simulink model "ML3phase"  (R2021a)
settings: Solver=VariableStepAuto  StartTime=0.0  StopTime=0.4  RelTol=1e-3
InitFcn:
  | alp1=30;
  | alp2=60;
values from neighbouring files (symbols this model uses):
  Alpha1 = z(1)    [ML3ph.m]
  Alpha2 = z(2)    [ML3ph.m]
  Alpha3 = z(3)    [ML3ph.m]
libraries: spsMosfetLib x36, spsCurrentMeasurementLib x10, spsDCVoltageSourceLib x9, spspowerguiLib x4, spsVoltageMeasurementLib x3, spsSeriesRLCBranchLib x3, spsGroundLib x1, spsRMSLib x1, spsThreePhaseVIMeasurementLib x1
settings Model: Creator=oem  LastModifiedBy=Islam
settings SolverCC: AlgebraicLoopSolver=TrustRegion
settings DataIOCC: SignalLogging=off  DSMLogging=off  ReturnWorkspaceOutputs=off
settings OptimizationCC: LifeSpan=inf
settings DebuggingCC: UnconnectedInputMsg=none  UnconnectedOutputMsg=none  UnconnectedLineMsg=none  SFMachineParentedDataDiag=warning  ArithmeticOperatorsInVariantConditions=warning
settings ModelReferenceCC: EnableRefExpFcnMdlSchedulingChecks=off
settings SFSimCC: CustomCodeUndefinedFunction=UseInterfaceOnly
settings RTWCC: Description=Generic Real-Time Target
settings CodeAppCC: StateflowObjectComments=on

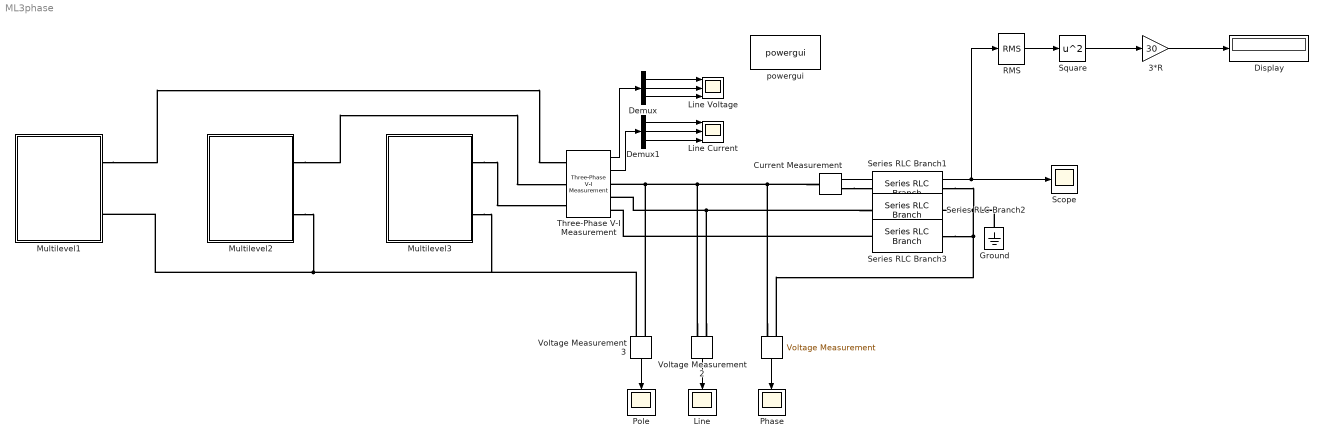
== system ML3phase ==
  " " : spsVoltageMeasurementLib/Voltage Measurement  PhasorSimulation=off  OutputType=Complex  PSBequivalent=0
  3*R : Gain  Gain=30
  Current Measurement : spsCurrentMeasurementLib/Current Measurement  PhasorSimulation=off  OutputType=Complex  PSBequivalent=0
  Demux : Demux  Outputs=3
  Demux1 : Demux  Outputs=3
  Display : Display
  Ground : spsGroundLib/Ground  LConnTagsString=a
  Line : Scope
  Line Current : Scope  NumInputPorts=3
  Line Voltage : Scope  NumInputPorts=3
  Multilevel1 : Subsystem
  Multilevel2 : Subsystem
  Multilevel3 : Subsystem
  Phase : Scope
  Pole : Scope
  RMS : spsRMSLib/RMS  TrueRMS=on  Freq=50  RMSInit=0  Ts=0
  Scope : Scope
  Series RLC Branch1 : spsSeriesRLCBranchLib/Series RLC Branch  LConnTagsString=__new0  RConnTagsString=__new0  BranchType=RL  Resistance=10  Inductance=1e-3  SetiL0=off  InitialCurrent=0  Capacitance=1e-6  Setx0=off  InitialVoltage=0  Measurements=None
  Series RLC Branch2 : spsSeriesRLCBranchLib/Series RLC Branch  LConnTagsString=__new0  RConnTagsString=__new0  BranchType=RL  Resistance=10  Inductance=1e-3  SetiL0=off  InitialCurrent=0  Capacitance=1e-6  Setx0=off  InitialVoltage=0  Measurements=None
  Series RLC Branch3 : spsSeriesRLCBranchLib/Series RLC Branch  LConnTagsString=__new0  RConnTagsString=__new0  BranchType=RL  Resistance=10  Inductance=1e-3  SetiL0=off  InitialCurrent=0  Capacitance=1e-6  Setx0=off  InitialVoltage=0  Measurements=None
  Square : Math  Operator=square  SaturateOnIntegerOverflow=on
  Three-Phase V-I Measurement : spsThreePhaseVIMeasurementLib/Three-Phase V-I Measurement  VoltageMeasurement=phase-to-phase  SetLabelV=off  LabelV=Vabc  Vpu=off  VpuLL=off  CurrentMeasurement=yes  SetLabelI=off  LabelI=Iabc  Ipu=off  Pbase=100e6  Vbase=500e3  OutputType=Complex  PhasorSimulation=off  PSBequivalent=0
  Voltage Measurement2 : spsVoltageMeasurementLib/Voltage Measurement  PhasorSimulation=off  OutputType=Complex  PSBequivalent=0
  Voltage Measurement3 : spsVoltageMeasurementLib/Voltage Measurement  PhasorSimulation=off  OutputType=Complex  PSBequivalent=0
  powergui : spspowerguiLib/powergui  Priority=1  SimulationMode=Continuous  SampleTime=50e-6  frequency=60  Iterations=50  frequencyindice=0  Pbase=100e6  ErrMax=1e-4  UnitsV=kV  UnitsW=MW  buscounter=0  FunctionMessages=off  echomessages=off  EnableUseOfTLC=off  CurrentSourceSwitches=off  DisableSnubberDevices=off  DisableRonSwitches=off  DisableVfSwitches=off  DisplayEquations=off  AutomaticDiscreteSolvers=off  SolverType=Tustin/Backward Euler (TBE)  Interpol=off  ExternalGateDelay=off  methode=off  Ts=100  x0status=blocks  SPID=on  SwTol=0  HookPort=off  NonlinearTolerance=1e-4  nMaxIteration=100  ContinueOnMaxIteration=off  RestoreLinks=warning  ResistiveCurrentMeasurement=off  Frange=[0:2:500]  Ylog=off  Xlog=on  ShowGrid=off  save=off  variable=ZData  structure=0  ZoomFFT=off  StartTime=0.0  cycles=1  DisplayStyle=1  fundamental=60  FreqAxis=off  MaxFrequency=1000  frequencyindicesteady=1  RmsSteady=1  display=off
  wires:
  Demux/3 -> Line Voltage/3
  Demux/1 -> Line Voltage/1
  Three-Phase V-I Measurement/1 -> Demux/1
  Demux/2 -> Line Voltage/2
  Demux1/1 -> Line Current/1
  Demux1/3 -> Line Current/3
  Three-Phase V-I Measurement/2 -> Demux1/1
  Demux1/2 -> Line Current/2
  " "/1 -> Phase/1
  Voltage Measurement2/1 -> Line/1
  Voltage Measurement3/1 -> Pole/1
  Current Measurement/1 -> RMS/1, Scope/1
  RMS/1 -> Square/1
  Square/1 -> 3*R/1
  3*R/1 -> Display/1
  connections:
  Multilevel2/RConn2 -- Voltage Measurement3/LConn2 -- Multilevel3/RConn2 -- Multilevel1/RConn2
  Multilevel3/RConn1 -- Three-Phase V-I Measurement/LConn3
  Multilevel2/RConn1 -- Three-Phase V-I Measurement/LConn2
  Multilevel1/RConn1 -- Three-Phase V-I Measurement/LConn1
  Series RLC Branch3/RConn1 -- Series RLC Branch2/RConn1 -- Series RLC Branch1/RConn1 -- Ground/LConn1 -- " "/LConn2
  " "/LConn1 -- Voltage Measurement2/LConn1 -- Voltage Measurement3/LConn1 -- Three-Phase V-I Measurement/RConn1 -- Current Measurement/LConn1
  Series RLC Branch2/LConn1 -- Voltage Measurement2/LConn2 -- Three-Phase V-I Measurement/RConn2
  Series RLC Branch3/LConn1 -- Three-Phase V-I Measurement/RConn3
  Current Measurement/RConn1 -- Series RLC Branch1/LConn1

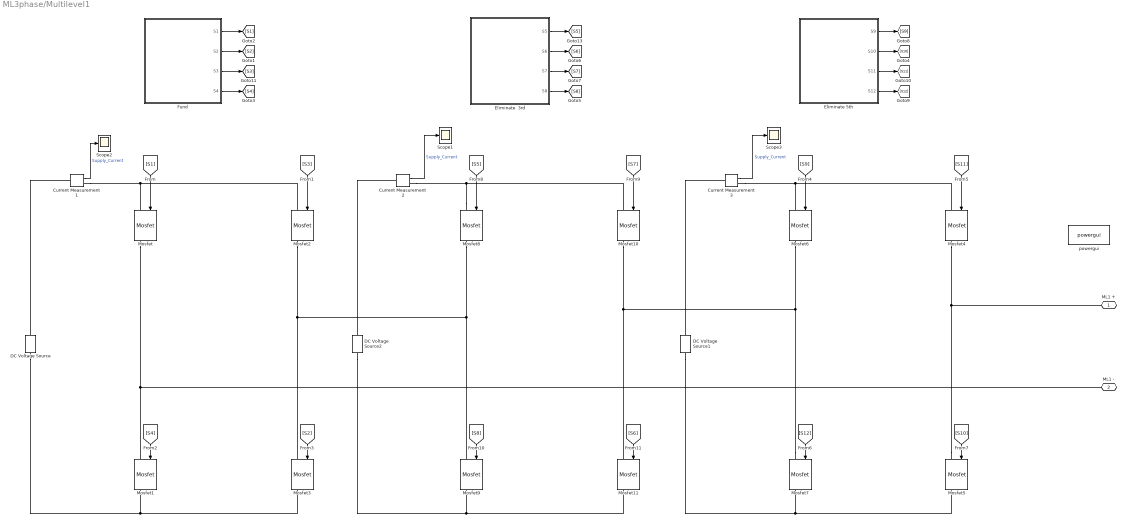
== system ML3phase/Multilevel1 ==
  Current Measurement1 : spsCurrentMeasurementLib/Current Measurement  PhasorSimulation=off  OutputType=Complex  PSBequivalent=0
  Current Measurement2 : spsCurrentMeasurementLib/Current Measurement  PhasorSimulation=off  OutputType=Complex  PSBequivalent=0
  Current Measurement3 : spsCurrentMeasurementLib/Current Measurement  PhasorSimulation=off  OutputType=Complex  PSBequivalent=0
  DC Voltage Source : spsDCVoltageSourceLib/DC Voltage Source  Amplitude=200/3  Measurements=Voltage
  DC Voltage Source1 : spsDCVoltageSourceLib/DC Voltage Source  Amplitude=200/3  Measurements=Voltage
  DC Voltage Source2 : spsDCVoltageSourceLib/DC Voltage Source  Amplitude=200/3  Measurements=Voltage
  Eliminate  3rd : Subsystem
  Eliminate 5th : Subsystem
  Fund : Subsystem
  Mosfet{,1..11} (12 alike) : spsMosfetLib/Mosfet  Ron=0.1  Lon=0  Rd=0.01  Vfd=0  IC=0  Rs=1e5  Cs=inf  Measurements=on
  Scope1 : Scope
  Scope2 : Scope
  Scope3 : Scope
  powergui : spspowerguiLib/powergui  Priority=1  SimulationMode=Continuous  SampleTime=1e-6  frequency=60  Iterations=50  frequencyindice=0  Pbase=100e6  ErrMax=1e-4  UnitsV=kV  UnitsW=MW  buscounter=0  FunctionMessages=off  echomessages=off  EnableUseOfTLC=off  CurrentSourceSwitches=off  DisableSnubberDevices=off  DisableRonSwitches=off  DisableVfSwitches=off  DisplayEquations=off  AutomaticDiscreteSolvers=off  SolverType=Tustin/Backward Euler (TBE)  Interpol=off  ExternalGateDelay=off  methode=off  Ts=100  x0status=blocks  SPID=on  SwTol=0  HookPort=off  NonlinearTolerance=1e-4  nMaxIteration=100  ContinueOnMaxIteration=off  RestoreLinks=warning  ResistiveCurrentMeasurement=off  Frange=[0:2:500]  Ylog=off  Xlog=on  ShowGrid=off  save=off  variable=ZData  structure=0  ZoomFFT=off  StartTime=0.0  cycles=1  DisplayStyle=1  fundamental=60  FreqAxis=off  MaxFrequency=1000  frequencyindicesteady=1  RmsSteady=1  display=off
  "ML1 + " : PMIOPort  Side=Right
  ML1 - : PMIOPort  Port=2  Side=Right
  wires:
  Eliminate 5th/1(S9) -> [S9]
  Fund/1(S1) -> [S1]
  [S8] -> Mosfet9/1
  [S1] -> Mosfet/1
  Eliminate  3rd/2(S6) -> [S6]
  [S12] -> Mosfet7/1
  [S11] -> Mosfet4/1
  Current Measurement3/1 -> Scope3/1  "Supply_Current"
  Eliminate 5th/2(S10) -> [S10]
  Fund/3(S3) -> [S3]
  [S2] -> Mosfet3/1
  Eliminate  3rd/1(S5) -> [S5]
  [S3] -> Mosfet2/1
  Current Measurement2/1 -> Scope1/1  "Supply_Current"
  Fund/2(S2) -> [S2]
  Current Measurement1/1 -> Scope2/1  "Supply_Current"
  [S4] -> Mosfet1/1
  [S5] -> Mosfet8/1
  [S6] -> Mosfet11/1
  Eliminate 5th/3(S11) -> [S11]
  Fund/4(S4) -> [S4]
  [S10] -> Mosfet5/1
  [S7] -> Mosfet10/1
  [S9] -> Mosfet6/1
  Eliminate  3rd/4(S8) -> [S8]
  Eliminate  3rd/3(S7) -> [S7]
  Eliminate 5th/4(S12) -> [S12]
  connections:
  Mosfet11/RConn1 -- DC Voltage Source2/LConn1 -- Mosfet9/RConn1
  Mosfet1/RConn1 -- Mosfet3/RConn1 -- DC Voltage Source/LConn1
  Mosfet8/LConn1 -- Current Measurement2/RConn1 -- Mosfet10/LConn1
  Mosfet5/LConn1 -- "ML1 + "/RConn1 -- Mosfet4/RConn1
  Current Measurement1/RConn1 -- Mosfet/LConn1 -- Mosfet2/LConn1
  Mosfet7/LConn1 -- Mosfet6/RConn1 -- Mosfet11/LConn1 -- Mosfet10/RConn1
  DC Voltage Source1/LConn1 -- Mosfet5/RConn1 -- Mosfet7/RConn1
  Mosfet/RConn1 -- Mosfet1/LConn1 -- ML1 -/RConn1
  Mosfet8/RConn1 -- Mosfet9/LConn1 -- Mosfet2/RConn1 -- Mosfet3/LConn1
  Current Measurement3/RConn1 -- Mosfet6/LConn1 -- Mosfet4/LConn1
  Current Measurement2/LConn1 -- DC Voltage Source2/RConn1
  Current Measurement3/LConn1 -- DC Voltage Source1/RConn1
  Current Measurement1/LConn1 -- DC Voltage Source/RConn1

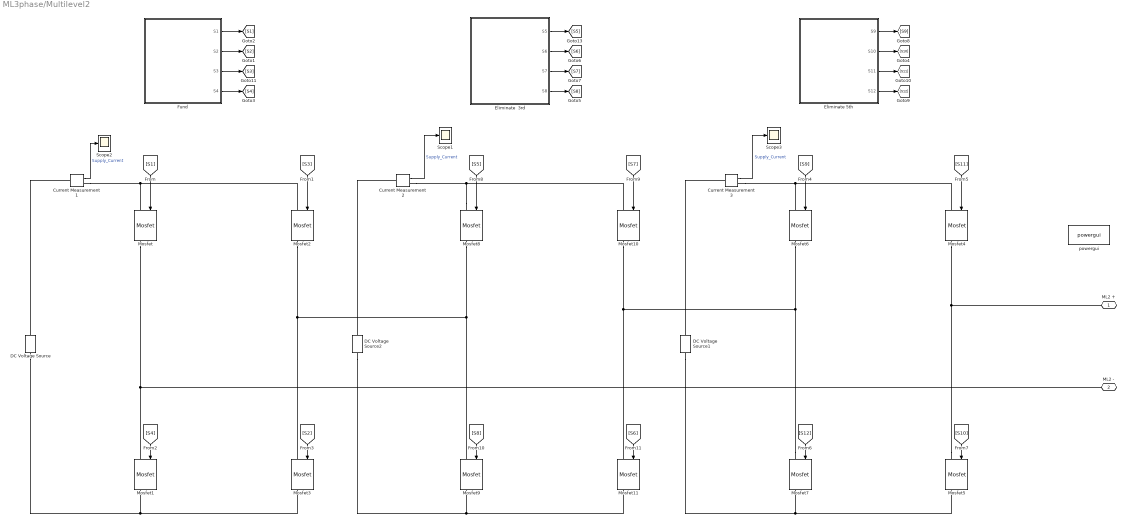
== system ML3phase/Multilevel2 ==
  Current Measurement1 : spsCurrentMeasurementLib/Current Measurement  PhasorSimulation=off  OutputType=Complex  PSBequivalent=0
  Current Measurement2 : spsCurrentMeasurementLib/Current Measurement  PhasorSimulation=off  OutputType=Complex  PSBequivalent=0
  Current Measurement3 : spsCurrentMeasurementLib/Current Measurement  PhasorSimulation=off  OutputType=Complex  PSBequivalent=0
  DC Voltage Source : spsDCVoltageSourceLib/DC Voltage Source  Amplitude=200/3  Measurements=Voltage
  DC Voltage Source1 : spsDCVoltageSourceLib/DC Voltage Source  Amplitude=200/3  Measurements=Voltage
  DC Voltage Source2 : spsDCVoltageSourceLib/DC Voltage Source  Amplitude=200/3  Measurements=Voltage
  Eliminate  3rd : Subsystem
  Eliminate 5th : Subsystem
  Fund : Subsystem
  Mosfet{,1..11} (12 alike) : spsMosfetLib/Mosfet  Ron=0.1  Lon=0  Rd=0.01  Vfd=0  IC=0  Rs=1e5  Cs=inf  Measurements=on
  Scope1 : Scope
  Scope2 : Scope
  Scope3 : Scope
  powergui : spspowerguiLib/powergui  Priority=1  SimulationMode=Continuous  SampleTime=1e-6  frequency=60  Iterations=50  frequencyindice=0  Pbase=100e6  ErrMax=1e-4  UnitsV=kV  UnitsW=MW  buscounter=0  FunctionMessages=off  echomessages=off  EnableUseOfTLC=off  CurrentSourceSwitches=off  DisableSnubberDevices=off  DisableRonSwitches=off  DisableVfSwitches=off  DisplayEquations=off  AutomaticDiscreteSolvers=off  SolverType=Tustin/Backward Euler (TBE)  Interpol=off  ExternalGateDelay=off  methode=off  Ts=100  x0status=blocks  SPID=on  SwTol=0  HookPort=off  NonlinearTolerance=1e-4  nMaxIteration=100  ContinueOnMaxIteration=off  RestoreLinks=warning  ResistiveCurrentMeasurement=off  Frange=[0:2:500]  Ylog=off  Xlog=on  ShowGrid=off  save=off  variable=ZData  structure=0  ZoomFFT=off  StartTime=0.0  cycles=1  DisplayStyle=1  fundamental=60  FreqAxis=off  MaxFrequency=1000  frequencyindicesteady=1  RmsSteady=1  display=off
  "ML2 + " : PMIOPort  Side=Right
  ML2 - : PMIOPort  Port=2  Side=Right
  wires:
  Eliminate 5th/1(S9) -> [S9]
  Fund/1(S1) -> [S1]
  [S8] -> Mosfet9/1
  [S1] -> Mosfet/1
  Eliminate  3rd/2(S6) -> [S6]
  [S12] -> Mosfet7/1
  [S11] -> Mosfet4/1
  Current Measurement3/1 -> Scope3/1  "Supply_Current"
  Eliminate 5th/2(S10) -> [S10]
  Fund/3(S3) -> [S3]
  [S2] -> Mosfet3/1
  Eliminate  3rd/1(S5) -> [S5]
  [S3] -> Mosfet2/1
  Current Measurement2/1 -> Scope1/1  "Supply_Current"
  Fund/2(S2) -> [S2]
  Current Measurement1/1 -> Scope2/1  "Supply_Current"
  [S4] -> Mosfet1/1
  [S5] -> Mosfet8/1
  [S6] -> Mosfet11/1
  Eliminate 5th/3(S11) -> [S11]
  Fund/4(S4) -> [S4]
  [S10] -> Mosfet5/1
  [S7] -> Mosfet10/1
  [S9] -> Mosfet6/1
  Eliminate  3rd/4(S8) -> [S8]
  Eliminate  3rd/3(S7) -> [S7]
  Eliminate 5th/4(S12) -> [S12]
  connections:
  Mosfet11/RConn1 -- DC Voltage Source2/LConn1 -- Mosfet9/RConn1
  Mosfet1/RConn1 -- Mosfet3/RConn1 -- DC Voltage Source/LConn1
  Mosfet8/LConn1 -- Current Measurement2/RConn1 -- Mosfet10/LConn1
  Mosfet5/LConn1 -- Mosfet4/RConn1 -- "ML2 + "/RConn1
  Current Measurement1/RConn1 -- Mosfet/LConn1 -- Mosfet2/LConn1
  Mosfet7/LConn1 -- Mosfet6/RConn1 -- Mosfet11/LConn1 -- Mosfet10/RConn1
  DC Voltage Source1/LConn1 -- Mosfet5/RConn1 -- Mosfet7/RConn1
  ML2 -/RConn1 -- Mosfet/RConn1 -- Mosfet1/LConn1
  Mosfet8/RConn1 -- Mosfet9/LConn1 -- Mosfet2/RConn1 -- Mosfet3/LConn1
  Current Measurement3/RConn1 -- Mosfet6/LConn1 -- Mosfet4/LConn1
  Current Measurement2/LConn1 -- DC Voltage Source2/RConn1
  Current Measurement3/LConn1 -- DC Voltage Source1/RConn1
  Current Measurement1/LConn1 -- DC Voltage Source/RConn1

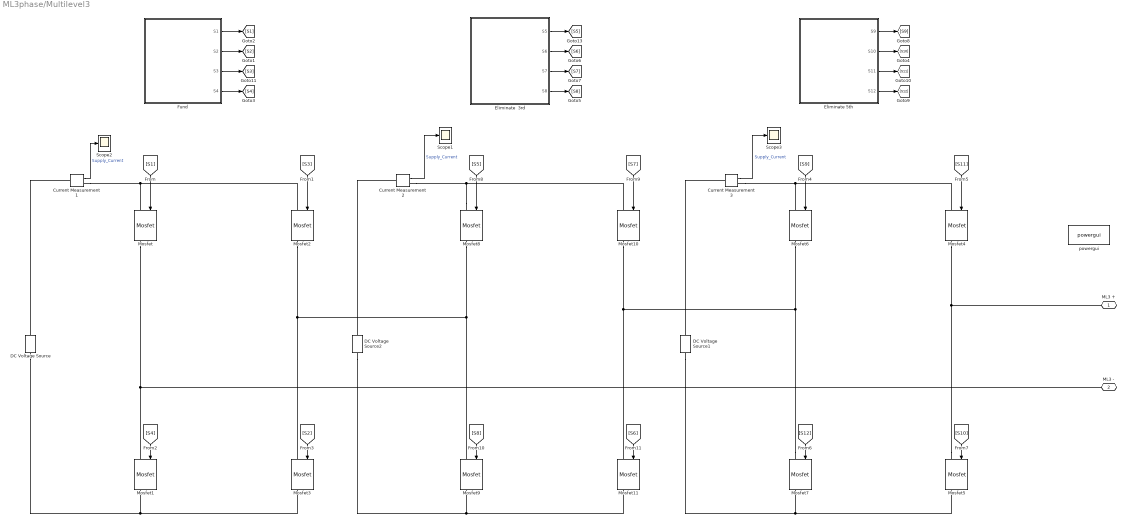
== system ML3phase/Multilevel3 ==
  Current Measurement1 : spsCurrentMeasurementLib/Current Measurement  PhasorSimulation=off  OutputType=Complex  PSBequivalent=0
  Current Measurement2 : spsCurrentMeasurementLib/Current Measurement  PhasorSimulation=off  OutputType=Complex  PSBequivalent=0
  Current Measurement3 : spsCurrentMeasurementLib/Current Measurement  PhasorSimulation=off  OutputType=Complex  PSBequivalent=0
  DC Voltage Source : spsDCVoltageSourceLib/DC Voltage Source  Amplitude=200/3  Measurements=Voltage
  DC Voltage Source1 : spsDCVoltageSourceLib/DC Voltage Source  Amplitude=200/3  Measurements=Voltage
  DC Voltage Source2 : spsDCVoltageSourceLib/DC Voltage Source  Amplitude=200/3  Measurements=Voltage
  Eliminate  3rd : Subsystem
  Eliminate 5th : Subsystem
  Fund : Subsystem
  Mosfet{,1..11} (12 alike) : spsMosfetLib/Mosfet  Ron=0.1  Lon=0  Rd=0.01  Vfd=0  IC=0  Rs=1e5  Cs=inf  Measurements=on
  Scope1 : Scope
  Scope2 : Scope
  Scope3 : Scope
  powergui : spspowerguiLib/powergui  Priority=1  SimulationMode=Continuous  SampleTime=1e-6  frequency=60  Iterations=50  frequencyindice=0  Pbase=100e6  ErrMax=1e-4  UnitsV=kV  UnitsW=MW  buscounter=0  FunctionMessages=off  echomessages=off  EnableUseOfTLC=off  CurrentSourceSwitches=off  DisableSnubberDevices=off  DisableRonSwitches=off  DisableVfSwitches=off  DisplayEquations=off  AutomaticDiscreteSolvers=off  SolverType=Tustin/Backward Euler (TBE)  Interpol=off  ExternalGateDelay=off  methode=off  Ts=100  x0status=blocks  SPID=on  SwTol=0  HookPort=off  NonlinearTolerance=1e-4  nMaxIteration=100  ContinueOnMaxIteration=off  RestoreLinks=warning  ResistiveCurrentMeasurement=off  Frange=[0:2:500]  Ylog=off  Xlog=on  ShowGrid=off  save=off  variable=ZData  structure=0  ZoomFFT=off  StartTime=0.0  cycles=1  DisplayStyle=1  fundamental=60  FreqAxis=off  MaxFrequency=1000  frequencyindicesteady=1  RmsSteady=1  display=off
  "ML3 + " : PMIOPort  Side=Right
  ML3 - : PMIOPort  Port=2  Side=Right
  wires:
  Eliminate 5th/1(S9) -> [S9]
  Fund/1(S1) -> [S1]
  [S8] -> Mosfet9/1
  [S1] -> Mosfet/1
  Eliminate  3rd/2(S6) -> [S6]
  [S12] -> Mosfet7/1
  [S11] -> Mosfet4/1
  Current Measurement3/1 -> Scope3/1  "Supply_Current"
  Eliminate 5th/2(S10) -> [S10]
  Fund/3(S3) -> [S3]
  [S2] -> Mosfet3/1
  Eliminate  3rd/1(S5) -> [S5]
  [S3] -> Mosfet2/1
  Current Measurement2/1 -> Scope1/1  "Supply_Current"
  Fund/2(S2) -> [S2]
  Current Measurement1/1 -> Scope2/1  "Supply_Current"
  [S4] -> Mosfet1/1
  [S5] -> Mosfet8/1
  [S6] -> Mosfet11/1
  Eliminate 5th/3(S11) -> [S11]
  Fund/4(S4) -> [S4]
  [S10] -> Mosfet5/1
  [S7] -> Mosfet10/1
  [S9] -> Mosfet6/1
  Eliminate  3rd/4(S8) -> [S8]
  Eliminate  3rd/3(S7) -> [S7]
  Eliminate 5th/4(S12) -> [S12]
  connections:
  Mosfet11/RConn1 -- DC Voltage Source2/LConn1 -- Mosfet9/RConn1
  Mosfet1/RConn1 -- Mosfet3/RConn1 -- DC Voltage Source/LConn1
  Mosfet8/LConn1 -- Current Measurement2/RConn1 -- Mosfet10/LConn1
  Mosfet5/LConn1 -- Mosfet4/RConn1 -- "ML3 + "/RConn1
  Current Measurement1/RConn1 -- Mosfet/LConn1 -- Mosfet2/LConn1
  Mosfet7/LConn1 -- Mosfet6/RConn1 -- Mosfet11/LConn1 -- Mosfet10/RConn1
  DC Voltage Source1/LConn1 -- Mosfet5/RConn1 -- Mosfet7/RConn1
  ML3 -/RConn1 -- Mosfet/RConn1 -- Mosfet1/LConn1
  Mosfet8/RConn1 -- Mosfet9/LConn1 -- Mosfet2/RConn1 -- Mosfet3/LConn1
  Current Measurement3/RConn1 -- Mosfet6/LConn1 -- Mosfet4/LConn1
  Current Measurement2/LConn1 -- DC Voltage Source2/RConn1
  Current Measurement3/LConn1 -- DC Voltage Source1/RConn1
  Current Measurement1/LConn1 -- DC Voltage Source/RConn1

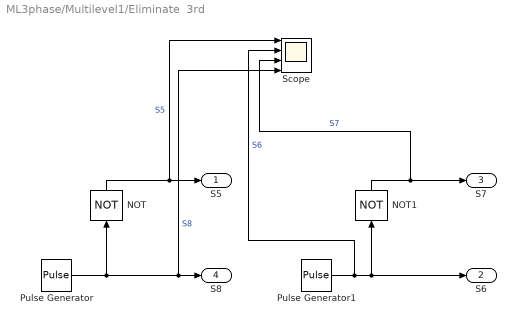
== system ML3phase/Multilevel1/Eliminate  3rd ==
  NOT : Logic  Operator=NOT  IconShape=distinctive  AllPortsSameDT=off  OutDataTypeStr=boolean
  NOT1 : Logic  Operator=NOT  IconShape=distinctive  AllPortsSameDT=off  OutDataTypeStr=boolean
  Pulse Generator : DiscretePulseGenerator  PulseType=Time based  Period=0.02  PulseWidth=(180-2*Alpha2)/360*100  PhaseDelay=(Alpha2/360)*0.02
  Pulse Generator1 : DiscretePulseGenerator  PulseType=Time based  Period=0.02  PulseWidth=(180-2*Alpha2)/360*100  PhaseDelay=0.01+((Alpha2/360)*0.02)
  Scope : Scope  NumInputPorts=4
  S5 : Outport
  S6 : Outport  Port=2
  S7 : Outport  Port=3
  S8 : Outport  Port=4
  wires:
  NOT/1 -> Scope/1, S5/1  "S5"
  Pulse Generator/1 -> NOT/1, Scope/4, S8/1  "S8"
  NOT1/1 -> Scope/3, S7/1  "S7"
  Pulse Generator1/1 -> Scope/2, NOT1/1, S6/1  "S6"

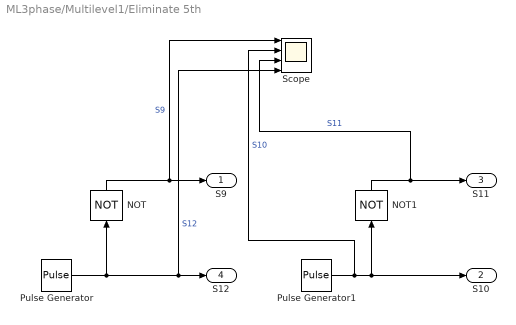
== system ML3phase/Multilevel1/Eliminate 5th ==
  NOT : Logic  Operator=NOT  IconShape=distinctive  AllPortsSameDT=off  OutDataTypeStr=boolean
  NOT1 : Logic  Operator=NOT  IconShape=distinctive  AllPortsSameDT=off  OutDataTypeStr=boolean
  Pulse Generator : DiscretePulseGenerator  PulseType=Time based  Period=0.02  PulseWidth=(180-2*Alpha3)/360*100  PhaseDelay=(Alpha3/360)*0.02
  Pulse Generator1 : DiscretePulseGenerator  PulseType=Time based  Period=0.02  PulseWidth=(180-2*Alpha3)/360*100  PhaseDelay=0.01+((Alpha3/360)*0.02)  VectorParams1D=off
  Scope : Scope  NumInputPorts=4
  S9 : Outport
  S10 : Outport  Port=2
  S11 : Outport  Port=3
  S12 : Outport  Port=4
  wires:
  Pulse Generator1/1 -> Scope/2, S10/1, NOT1/1  "S10"
  NOT1/1 -> Scope/3, S11/1  "S11"
  Pulse Generator/1 -> Scope/4, S12/1, NOT/1  "S12"
  NOT/1 -> Scope/1, S9/1  "S9"

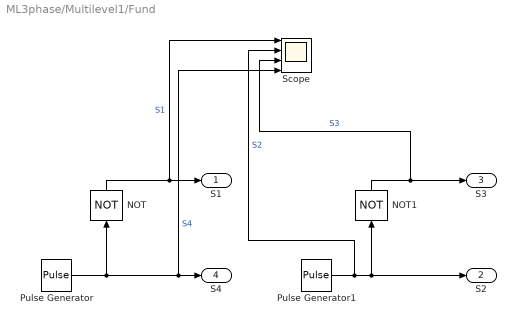
== system ML3phase/Multilevel1/Fund ==
  NOT : Logic  Operator=NOT  IconShape=distinctive  AllPortsSameDT=off  OutDataTypeStr=boolean
  NOT1 : Logic  Operator=NOT  IconShape=distinctive  AllPortsSameDT=off  OutDataTypeStr=boolean
  Pulse Generator : DiscretePulseGenerator  PulseType=Time based  Period=0.02  PulseWidth=(180-2*Alpha1)/360*100  PhaseDelay=(Alpha1/360)*0.02
  Pulse Generator1 : DiscretePulseGenerator  PulseType=Time based  Period=0.02  PulseWidth=(180-2*Alpha1)/360*100  PhaseDelay=0.01+((Alpha1/360)*0.02)
  Scope : Scope  NumInputPorts=4
  S1 : Outport
  S2 : Outport  Port=2
  S3 : Outport  Port=3
  S4 : Outport  Port=4
  wires:
  NOT/1 -> Scope/1, S1/1  "S1"
  Pulse Generator/1 -> NOT/1, Scope/4, S4/1  "S4"
  NOT1/1 -> Scope/3, S3/1  "S3"
  Pulse Generator1/1 -> Scope/2, NOT1/1, S2/1  "S2"

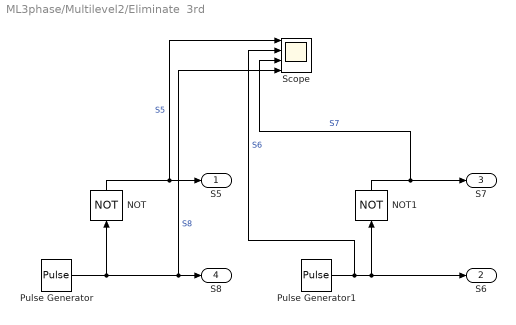
== system ML3phase/Multilevel2/Eliminate  3rd ==
  NOT : Logic  Operator=NOT  IconShape=distinctive  AllPortsSameDT=off  OutDataTypeStr=boolean
  NOT1 : Logic  Operator=NOT  IconShape=distinctive  AllPortsSameDT=off  OutDataTypeStr=boolean
  Pulse Generator : DiscretePulseGenerator  PulseType=Time based  Period=0.02  PulseWidth=(180-2*Alpha2)/360*100  PhaseDelay=1/150+(Alpha2/360)*0.02
  Pulse Generator1 : DiscretePulseGenerator  PulseType=Time based  Period=0.02  PulseWidth=(180-2*Alpha2)/360*100  PhaseDelay=1/60+((Alpha2/360)*0.02)
  Scope : Scope  NumInputPorts=4
  S5 : Outport
  S6 : Outport  Port=2
  S7 : Outport  Port=3
  S8 : Outport  Port=4
  wires:
  NOT/1 -> Scope/1, S5/1  "S5"
  Pulse Generator/1 -> NOT/1, Scope/4, S8/1  "S8"
  NOT1/1 -> Scope/3, S7/1  "S7"
  Pulse Generator1/1 -> Scope/2, NOT1/1, S6/1  "S6"

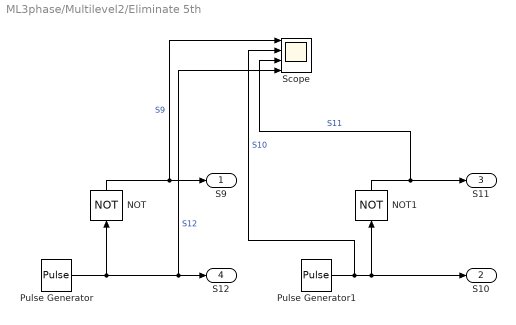
== system ML3phase/Multilevel2/Eliminate 5th ==
  NOT : Logic  Operator=NOT  IconShape=distinctive  AllPortsSameDT=off  OutDataTypeStr=boolean
  NOT1 : Logic  Operator=NOT  IconShape=distinctive  AllPortsSameDT=off  OutDataTypeStr=boolean
  Pulse Generator : DiscretePulseGenerator  PulseType=Time based  Period=0.02  PulseWidth=(180-2*Alpha3)/360*100  PhaseDelay=1/150+(Alpha3/360)*0.02
  Pulse Generator1 : DiscretePulseGenerator  PulseType=Time based  Period=0.02  PulseWidth=(180-2*Alpha3)/360*100  PhaseDelay=1/60+((Alpha3/360)*0.02)  VectorParams1D=off
  Scope : Scope  NumInputPorts=4
  S9 : Outport
  S10 : Outport  Port=2
  S11 : Outport  Port=3
  S12 : Outport  Port=4
  wires:
  Pulse Generator1/1 -> Scope/2, S10/1, NOT1/1  "S10"
  NOT1/1 -> Scope/3, S11/1  "S11"
  Pulse Generator/1 -> Scope/4, S12/1, NOT/1  "S12"
  NOT/1 -> Scope/1, S9/1  "S9"

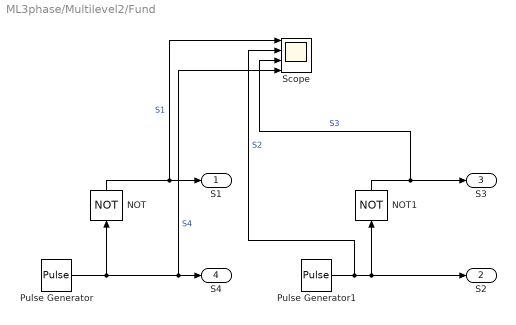
== system ML3phase/Multilevel2/Fund ==
  NOT : Logic  Operator=NOT  IconShape=distinctive  AllPortsSameDT=off  OutDataTypeStr=boolean
  NOT1 : Logic  Operator=NOT  IconShape=distinctive  AllPortsSameDT=off  OutDataTypeStr=boolean
  Pulse Generator : DiscretePulseGenerator  PulseType=Time based  Period=0.02  PulseWidth=(180-2*Alpha1)/360*100  PhaseDelay=1/150+(Alpha1/360)*0.02
  Pulse Generator1 : DiscretePulseGenerator  PulseType=Time based  Period=0.02  PulseWidth=(180-2*Alpha1)/360*100  PhaseDelay=1/60+((Alpha1/360)*0.02)
  Scope : Scope  NumInputPorts=4
  S1 : Outport
  S2 : Outport  Port=2
  S3 : Outport  Port=3
  S4 : Outport  Port=4
  wires:
  NOT/1 -> Scope/1, S1/1  "S1"
  Pulse Generator/1 -> NOT/1, Scope/4, S4/1  "S4"
  NOT1/1 -> Scope/3, S3/1  "S3"
  Pulse Generator1/1 -> Scope/2, NOT1/1, S2/1  "S2"

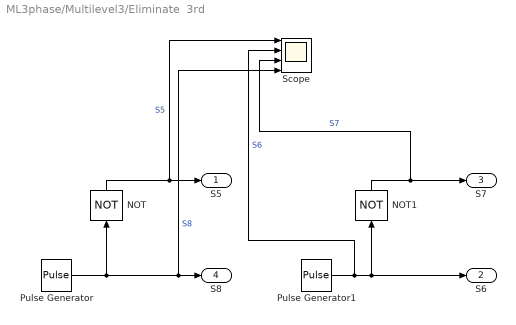
== system ML3phase/Multilevel3/Eliminate  3rd ==
  NOT : Logic  Operator=NOT  IconShape=distinctive  AllPortsSameDT=off  OutDataTypeStr=boolean
  NOT1 : Logic  Operator=NOT  IconShape=distinctive  AllPortsSameDT=off  OutDataTypeStr=boolean
  Pulse Generator : DiscretePulseGenerator  PulseType=Time based  Period=0.02  PulseWidth=(180-2*Alpha2)/360*100  PhaseDelay=1/75+(Alpha2/360)*0.02
  Pulse Generator1 : DiscretePulseGenerator  PulseType=Time based  Period=0.02  PulseWidth=(180-2*Alpha2)/360*100  PhaseDelay=7/300+((Alpha2/360)*0.02)
  Scope : Scope  NumInputPorts=4
  S5 : Outport
  S6 : Outport  Port=2
  S7 : Outport  Port=3
  S8 : Outport  Port=4
  wires:
  NOT/1 -> Scope/1, S5/1  "S5"
  Pulse Generator/1 -> NOT/1, Scope/4, S8/1  "S8"
  NOT1/1 -> Scope/3, S7/1  "S7"
  Pulse Generator1/1 -> Scope/2, NOT1/1, S6/1  "S6"

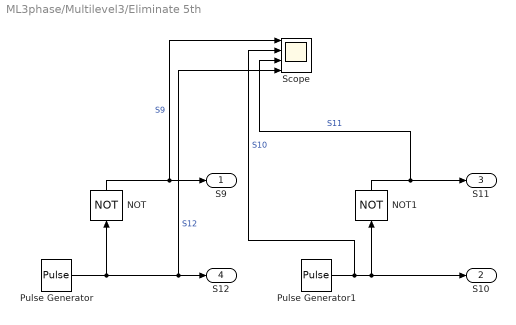
== system ML3phase/Multilevel3/Eliminate 5th ==
  NOT : Logic  Operator=NOT  IconShape=distinctive  AllPortsSameDT=off  OutDataTypeStr=boolean
  NOT1 : Logic  Operator=NOT  IconShape=distinctive  AllPortsSameDT=off  OutDataTypeStr=boolean
  Pulse Generator : DiscretePulseGenerator  PulseType=Time based  Period=0.02  PulseWidth=(180-2*Alpha3)/360*100  PhaseDelay=1/75+(Alpha3/360)*0.02
  Pulse Generator1 : DiscretePulseGenerator  PulseType=Time based  Period=0.02  PulseWidth=(180-2*Alpha3)/360*100  PhaseDelay=7/300+((Alpha3/360)*0.02)  VectorParams1D=off
  Scope : Scope  NumInputPorts=4
  S9 : Outport
  S10 : Outport  Port=2
  S11 : Outport  Port=3
  S12 : Outport  Port=4
  wires:
  Pulse Generator1/1 -> Scope/2, S10/1, NOT1/1  "S10"
  NOT1/1 -> Scope/3, S11/1  "S11"
  Pulse Generator/1 -> Scope/4, S12/1, NOT/1  "S12"
  NOT/1 -> Scope/1, S9/1  "S9"

== system ML3phase/Multilevel3/Fund ==
  NOT : Logic  Operator=NOT  IconShape=distinctive  AllPortsSameDT=off  OutDataTypeStr=boolean
  NOT1 : Logic  Operator=NOT  IconShape=distinctive  AllPortsSameDT=off  OutDataTypeStr=boolean
  Pulse Generator : DiscretePulseGenerator  PulseType=Time based  Period=0.02  PulseWidth=(180-2*Alpha1)/360*100  PhaseDelay=1/75+(Alpha1/360)*0.02
  Pulse Generator1 : DiscretePulseGenerator  PulseType=Time based  Period=0.02  PulseWidth=(180-2*Alpha1)/360*100  PhaseDelay=7/300+((Alpha1/360)*0.02)
  Scope : Scope  NumInputPorts=4
  S1 : Outport
  S2 : Outport  Port=2
  S3 : Outport  Port=3
  S4 : Outport  Port=4
  wires:
  NOT/1 -> Scope/1, S1/1  "S1"
  Pulse Generator/1 -> NOT/1, Scope/4, S4/1  "S4"
  NOT1/1 -> Scope/3, S3/1  "S3"
  Pulse Generator1/1 -> Scope/2, NOT1/1, S2/1  "S2"
